simulink model "Simulink_Simulation"  (Simulink 10.1)
settings: Solver=ode23t  StartTime=0.0  StopTime=0.08  RelTol=1e-3  EnableMultiTasking=on
libraries: powerlib x29, powerlib_meascontrol x4
settings Model: Creator=asus1  LastModifiedBy=x64
settings DataIOCC: LimitDataPoints=on
settings DebuggingCC: UnderspecifiedInitializationDetection=Simplified  MergeDetectMultiDrivingBlocksExec=error  SolverPrmCheckMsg=warning
settings GRTTargetCC: CombineOutputUpdateFcns=on  GRTInterface=off
settings ConfigComp: CovSFcnEnable=off
settings SimscapeCC: SimscapeNormalizeSystem=off

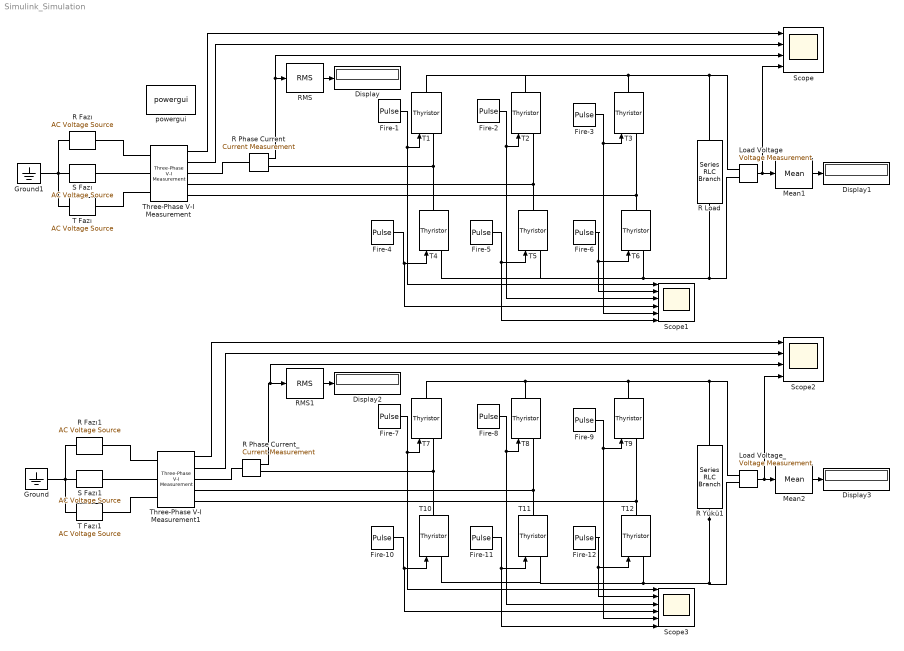
== system Simulink_Simulation ==
  Display{,1..3} (4 alike) : Display
      settings: Format=bank
  Fire-1 : DiscretePulseGenerator  PulseType=Time based  Period=0.02  PulseWidth=5  PhaseDelay=0.0033  VectorParams1D=off
  Fire-10 : DiscretePulseGenerator  PulseType=Time based  Period=0.02  PulseWidth=25  PhaseDelay=0.0167  VectorParams1D=off
  Fire-11 : DiscretePulseGenerator  PulseType=Time based  Period=0.02  PulseWidth=25  PhaseDelay=0.0233  VectorParams1D=off
  Fire-12 : DiscretePulseGenerator  PulseType=Time based  Period=0.02  PulseWidth=25  PhaseDelay=0.01  VectorParams1D=off
  Fire-2 : DiscretePulseGenerator  PulseType=Time based  Period=0.02  PulseWidth=5  PhaseDelay=0.01  VectorParams1D=off
  Fire-3 : DiscretePulseGenerator  PulseType=Time based  Period=0.02  PulseWidth=5  PhaseDelay=0.0167  VectorParams1D=off
  Fire-4 : DiscretePulseGenerator  PulseType=Time based  Period=0.02  PulseWidth=5  PhaseDelay=0.0133  VectorParams1D=off
  Fire-5 : DiscretePulseGenerator  PulseType=Time based  Period=0.02  PulseWidth=5  PhaseDelay=0.02  VectorParams1D=off
  Fire-6 : DiscretePulseGenerator  PulseType=Time based  Period=0.02  PulseWidth=5  PhaseDelay=0.0067  VectorParams1D=off
  Fire-7 : DiscretePulseGenerator  PulseType=Time based  Period=0.02  PulseWidth=25  PhaseDelay=0.0067  VectorParams1D=off
  Fire-8 : DiscretePulseGenerator  PulseType=Time based  Period=0.02  PulseWidth=25  PhaseDelay=0.0133  VectorParams1D=off
  Fire-9 : DiscretePulseGenerator  PulseType=Time based  Period=0.02  PulseWidth=25  PhaseDelay=0.02  VectorParams1D=off
  Ground : powerlib/Elements/Ground  LConnTagsString=a
  Ground1 : powerlib/Elements/Ground  LConnTagsString=a
  "Load Voltage " : powerlib/Measurements/Voltage Measurement  PhasorSimulation=off  OutputType=Complex  PSBequivalent=0
  Load Voltage_ : powerlib/Measurements/Voltage Measurement  PhasorSimulation=off  OutputType=Complex  PSBequivalent=0
  Mean1 : powerlib_meascontrol/Measurements/Mean  Freq=50  Vinit=0  Ts=0
  Mean2 : powerlib_meascontrol/Measurements/Mean  Freq=50  Vinit=0  Ts=0
  R Fazı : powerlib/Electrical Sources/AC Voltage Source  Amplitude=220*sqrt(2)  Phase=0  Frequency=50  SampleTime=0  Measurements=None  BusType=swing  Pref=10e3  Qref=0  Qmin=-inf  Qmax=+inf
  R Fazı1 : powerlib/Electrical Sources/AC Voltage Source  Amplitude=220*sqrt(2)  Phase=0  Frequency=50  SampleTime=0  Measurements=None  BusType=swing  Pref=10e3  Qref=0  Qmin=-inf  Qmax=+inf
  R Load : powerlib/Elements/Series RLC Branch  LConnTagsString=__new0  RConnTagsString=__new0  BranchType=R  Resistance=10  Inductance=1e-3  SetiL0=off  InitialCurrent=0  Capacitance=1e-6  Setx0=off  InitialVoltage=0  Measurements=None
  R Phase Current : powerlib/Measurements/Current Measurement  PhasorSimulation=off  OutputType=Complex  PSBequivalent=0
  R Phase Current_ : powerlib/Measurements/Current Measurement  PhasorSimulation=off  OutputType=Complex  PSBequivalent=0
  R Yükü1 : powerlib/Elements/Series RLC Branch  LConnTagsString=__new0  RConnTagsString=__new0  BranchType=R  Resistance=10  Inductance=1e-3  SetiL0=off  InitialCurrent=0  Capacitance=1e-6  Setx0=off  InitialVoltage=0  Measurements=None
  RMS : powerlib_meascontrol/Measurements/RMS  TrueRMS=on  Freq=50  RMSInit=0  Ts=0
  RMS1 : powerlib_meascontrol/Measurements/RMS  TrueRMS=on  Freq=50  RMSInit=0  Ts=0
  S Fazı : powerlib/Electrical Sources/AC Voltage Source  Amplitude=220*sqrt(2)  Phase=-120  Frequency=50  SampleTime=0  Measurements=None  BusType=swing  Pref=10e3  Qref=0  Qmin=-inf  Qmax=+inf
  S Fazı1 : powerlib/Electrical Sources/AC Voltage Source  Amplitude=220*sqrt(2)  Phase=-120  Frequency=50  SampleTime=0  Measurements=None  BusType=swing  Pref=10e3  Qref=0  Qmin=-inf  Qmax=+inf
  Scope : Scope  NumInputPorts=4
  Scope1 : Scope  NumInputPorts=6
  Scope2 : Scope  NumInputPorts=4
  Scope3 : Scope  NumInputPorts=6
  T Fazı : powerlib/Electrical Sources/AC Voltage Source  Amplitude=220*sqrt(2)  Phase=120  Frequency=50  SampleTime=0  Measurements=None  BusType=swing  Pref=10e3  Qref=0  Qmin=-inf  Qmax=+inf
  T Fazı1 : powerlib/Electrical Sources/AC Voltage Source  Amplitude=220*sqrt(2)  Phase=120  Frequency=50  SampleTime=0  Measurements=None  BusType=swing  Pref=10e3  Qref=0  Qmin=-inf  Qmax=+inf
  T{1..12} (12 alike) : powerlib/Power Electronics/Thyristor  Ron=0.0000001  Lon=0  Vf=0  IC=0  Rs=5000  Cs=250e-9  Measurements=off
  "Three-Phase V-I Measurement " : powerlib/Measurements/Three-Phase V-I Measurement  VoltageMeasurement=phase-to-ground  SetLabelV=off  LabelV=Vabc  Vpu=off  VpuLL=off  CurrentMeasurement=yes  SetLabelI=off  LabelI=Iabc  Ipu=off  Pbase=100e6  Vbase=500e3  OutputType=Complex  PhasorSimulation=off  PSBequivalent=0
  Three-Phase V-I Measurement1 : powerlib/Measurements/Three-Phase V-I Measurement  VoltageMeasurement=phase-to-ground  SetLabelV=off  LabelV=Vabc  Vpu=off  VpuLL=off  CurrentMeasurement=yes  SetLabelI=off  LabelI=Iabc  Ipu=off  Pbase=100e6  Vbase=500e3  OutputType=Complex  PhasorSimulation=off  PSBequivalent=0
  powergui : powerlib/powergui  Priority=1  SimulationMode=Discrete  SampleTime=5e-6  frequency=60  Iterations=50  frequencyindice=50  Pbase=100e6  ErrMax=1e-4  UnitsV=kV  UnitsW=MW  buscounter=0  FunctionMessages=off  echomessages=off  EnableUseOfTLC=off  CurrentSourceSwitches=off  DisableSnubberDevices=off  DisableRonSwitches=off  DisableVfSwitches=off  DisplayEquations=off  AutomaticDiscreteSolvers=off  SolverType=Tustin  Interpol=off  ExternalGateDelay=off  methode=off  Ts=100  x0status=blocks  SPID=off  SwTol=0  HookPort=off  NonlinearTolerance=1e-4  nMaxIteration=100  ContinueOnMaxIteration=off  RestoreLinks=warning  ResistiveCurrentMeasurement=off  Frange=[0:2:500]  Ylog=off  Xlog=on  ShowGrid=off  save=off  variable=ZData  structure=0  ZoomFFT=off  StartTime=0.0  cycles=1  DisplayStyle=1  fundamental=60  FreqAxis=off  MaxFrequency=1000  frequencyindicesteady=1  RmsSteady=1  display=off
  wires:
  "Load Voltage "/1 -> Scope/4, Mean1/1
  R Phase Current/1 -> Scope/3, RMS/1
  RMS/1 -> Display/1
  Mean1/1 -> Display1/1
  Fire-2/1 -> Scope1/3, T2/1
  Fire-3/1 -> Scope1/5, T3/1
  Fire-4/1 -> Scope1/4, T4/1
  Fire-5/1 -> Scope1/6, T5/1
  Fire-6/1 -> Scope1/2, T6/1
  Fire-1/1 -> Scope1/1, T1/1
  Load Voltage_/1 -> Scope2/4, Mean2/1
  R Phase Current_/1 -> Scope2/3, RMS1/1
  RMS1/1 -> Display2/1
  Mean2/1 -> Display3/1
  Fire-8/1 -> Scope3/3, T8/1
  Fire-9/1 -> Scope3/5, T9/1
  Fire-10/1 -> Scope3/4, T10/1
  Fire-11/1 -> Scope3/6, T11/1
  Fire-12/1 -> Scope3/2, T12/1
  Fire-7/1 -> Scope3/1, T7/1
  "Three-Phase V-I Measurement "/1 -> Scope/1
  "Three-Phase V-I Measurement "/2 -> Scope/2
  Three-Phase V-I Measurement1/1 -> Scope2/1
  Three-Phase V-I Measurement1/2 -> Scope2/2
  connections:
  T3/RConn1 -- T1/RConn1 -- T2/RConn1 -- "Load Voltage "/LConn1 -- R Load/LConn1
  R Phase Current/RConn1 -- T4/RConn1 -- T1/LConn1
  T6/RConn1 -- "Three-Phase V-I Measurement "/RConn3 -- T3/LConn1
  "Load Voltage "/LConn2 -- T5/LConn1 -- T4/LConn1 -- T6/LConn1 -- R Load/RConn1
  T8/RConn1 -- T7/RConn1 -- T9/RConn1 -- Load Voltage_/LConn1 -- R Yükü1/LConn1
  R Phase Current_/RConn1 -- T7/LConn1 -- T10/RConn1
  T11/RConn1 -- Three-Phase V-I Measurement1/RConn2 -- T8/LConn1
  T12/RConn1 -- T9/LConn1 -- Three-Phase V-I Measurement1/RConn3
  R Yükü1/RConn1 -- Load Voltage_/LConn2 -- T10/LConn1 -- T11/LConn1 -- T12/LConn1
  T5/RConn1 -- "Three-Phase V-I Measurement "/RConn2 -- T2/LConn1
  "Three-Phase V-I Measurement "/LConn2 -- S Fazı/RConn1
  R Fazı/RConn1 -- "Three-Phase V-I Measurement "/LConn1
  T Fazı/RConn1 -- "Three-Phase V-I Measurement "/LConn3
  T Fazı/LConn1 -- Ground1/LConn1 -- R Fazı/LConn1 -- S Fazı/LConn1
  "Three-Phase V-I Measurement "/RConn1 -- R Phase Current/LConn1
  Three-Phase V-I Measurement1/LConn2 -- S Fazı1/RConn1
  R Fazı1/RConn1 -- Three-Phase V-I Measurement1/LConn1
  T Fazı1/RConn1 -- Three-Phase V-I Measurement1/LConn3
  Three-Phase V-I Measurement1/RConn1 -- R Phase Current_/LConn1
  Ground/LConn1 -- S Fazı1/LConn1 -- R Fazı1/LConn1 -- T Fazı1/LConn1
